simulink library "db_tetha1"  (R2018a)
settings: Solver=VariableStepAuto  StartTime=0.0  StopTime=10.0  RelTol=1e-3
values from neighbouring files (symbols this model uses):
  B1 = 40    [ejemplo_mecanico.m]    (also in veengranes.m = 10)
  B2 = 20    [ejemplo_mecanico.m]    (also in veengranes.m = 34)
  J1 = 200    [Problem_5_Matlab.m]    (also in grupo_roberto.m = 3; veengranes.m = 2)
  J2 = 10    [Problem_5_Matlab.m]    (also in grupo_roberto.m = 3; veengranes.m = 4)
  K1 = 700    [Problem_5_Matlab.m]    (also in ejemplo_mecanico.m = 100; ejercicio7_taller2SM.m = 34; grupo_roberto.m = 3; veengranes.m = 5)
  K2 = 20    [Problem_5_Matlab.m]    (also in ejercicio7_taller2SM.m = 300; grupo_roberto.m = 3; veengranes.m = 4)
  r1 = 0.5    [veengranes.m]
  r2 = 0.1    [veengranes.m]
settings Model: Creator=carma  LastModifiedBy=carma

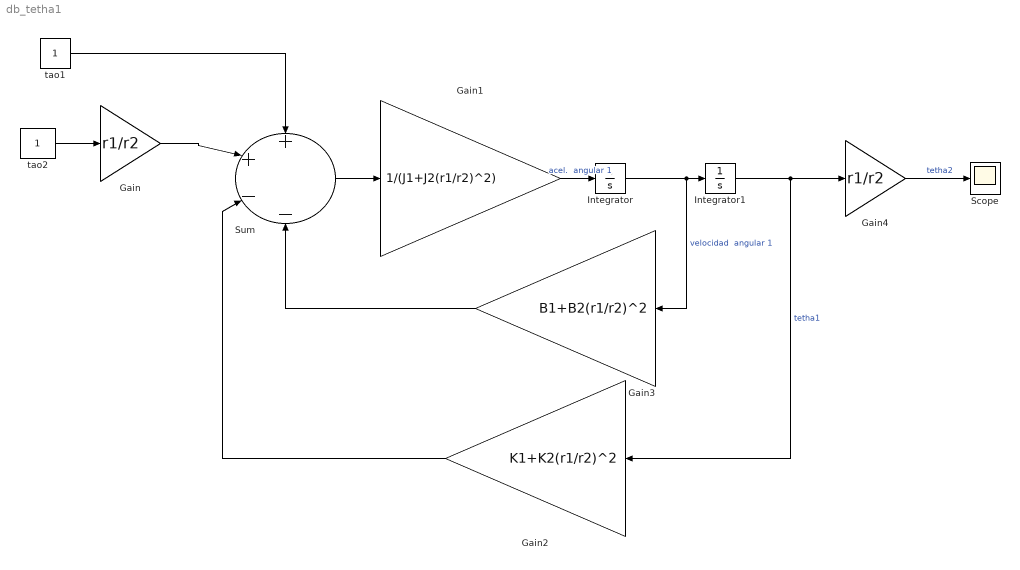
== system db_tetha1 ==
  Gain : Gain  Gain=r1/r2
  Gain1 : Gain  Gain=1/(J1+J2(r1/r2)^2)
  Gain2 : Gain  Gain=K1+K2(r1/r2)^2
  Gain3 : Gain  Gain=B1+B2(r1/r2)^2
  Gain4 : Gain  Gain=r1/r2
  Integrator : Integrator
  Integrator1 : Integrator
  Scope : Scope
  Sum : Sum  Inputs=++--
  tao1 : Constant
  tao2 : Constant
  wires:
  tao1/1 -> Sum/1
  tao2/1 -> Gain/1
  Gain/1 -> Sum/2
  Sum/1 -> Gain1/1
  Gain1/1 -> Integrator/1  "acel.  angular 1"
  Integrator/1 -> Gain3/1, Integrator1/1  "velocidad  angular 1"
  Integrator1/1 -> Gain2/1, Gain4/1  "tetha1"
  Gain2/1 -> Sum/3
  Gain3/1 -> Sum/4
  Gain4/1 -> Scope/1  "tetha2"
